simulink model "pendel1"  (Simulink 4.00)
settings: Solver=ode45  StartTime=0.0  StopTime=10.0  RelTol=1e-3
values from neighbouring files (symbols this model uses):
  g = 9.81    [behaelter_1.m]    (also in behaelter_2.m; kette_1.m = 9.8; pendel_1.m = 9.8; pendel_2.m = 9.8)
  l = 1    [pendel_1.m]
  m = 1    [pendel_1.m]    (also in pendel_2.m = 500)
  r = 2    [behaelter_1.m]    (also in behaelter_2.m; mehrw_1.m = [0.05, 0.05, 0.05, 0.05, 0.05]; mehrw_2.m = [0.05, 0.05, 0.05, 0.05, 0.05]; mehrw_3.m = [0.05, 0.05, 0.05, 0.05, 0.05])
  theta0 = 45*pi/180    (= 0.785398163397)    [pendel_1.m]    (also in pendel_2.m = 0.349065850399)
settings Model: LastModifiedBy=Administrator  BlockReductionOpt=off

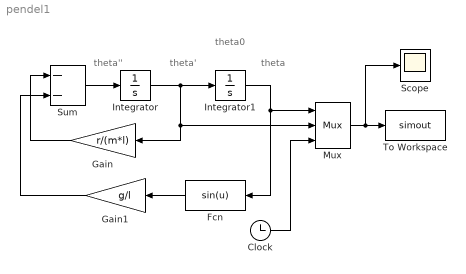
== system pendel1 ==
  note: theta''
  note: theta'
  note: theta
  note: theta0
  Clock : Clock
      settings: DisplayTime=off  Decimation=10
  Fcn : Fcn  Orientation=left  Expr=sin(u)
  Gain : Gain  Orientation=left  Gain=r/(m*l)  Multiplication=Element-wise(K.*u)  SaturateOnIntegerOverflow=on
  Gain1 : Gain  Orientation=left  Gain=g/l  Multiplication=Element-wise(K.*u)  SaturateOnIntegerOverflow=on
  Integrator : Integrator  ExternalReset=none  InitialConditionSource=internal  InitialCondition=0  LimitOutput=off  UpperSaturationLimit=inf  LowerSaturationLimit=-inf  ShowSaturationPort=off  ShowStatePort=off  AbsoluteTolerance=auto
  Integrator1 : Integrator  ExternalReset=none  InitialConditionSource=internal  InitialCondition=theta0  LimitOutput=off  UpperSaturationLimit=inf  LowerSaturationLimit=-inf  ShowSaturationPort=off  ShowStatePort=off  AbsoluteTolerance=auto
  Mux : Mux  Inputs=3
      settings: DisplayOption=none
  Scope : Scope
      settings: TimeRange=auto  YMin=-5  YMax=5  SaveToWorkspace=off  SaveName=ScopeData  LimitDataPoints=on  MaxDataPoints=5000
  Sum : Sum  Inputs=--  SaturateOnIntegerOverflow=on
  To Workspace : ToWorkspace  VariableName=simout  SampleTime=-1  SaveFormat=Array
  wires:
  Sum/1 -> Integrator/1
  Integrator/1 -> Integrator1/1, Gain/1, Mux/2
  Gain/1 -> Sum/1
  Gain1/1 -> Sum/2
  Integrator1/1 -> Fcn/1, Mux/1
  Fcn/1 -> Gain1/1
  Clock/1 -> Mux/3
  Mux/1 -> To Workspace/1, Scope/1
